simulink model "HevP2PowertrainController"  (R2022a)
settings: Solver=FixedStepDiscrete  StartTime=0  StopTime=inf  FixedStep=0.01  RelTol=1e-3  EnableMultiTasking=on
model workspace (MAT data in the model file):
  BattChargeMax = Simulink.Parameter
  BattChargeMax.Value = 5.3
  BattChargeMax.DataType = 'double'
  BattChargeMax.Complexity = 'real'
  BattChargeMax.Dimensions = [1 1]
  BattChrgPwrMax = Simulink.Parameter
  BattChrgPwrMax.Value = -30000
  BattChrgPwrMax.DataType = 'double'
  BattChrgPwrMax.Complexity = 'real'
  BattChrgPwrMax.Dimensions = [1 1]
  BattDischrgPwrMax = Simulink.Parameter
  BattDischrgPwrMax.Value = 46000
  BattDischrgPwrMax.DataType = 'double'
  BattDischrgPwrMax.Complexity = 'real'
  BattDischrgPwrMax.Dimensions = [1 1]
  BattEnrgy = Simulink.Parameter
  BattEnrgy.Value = 5724000
  BattEnrgy.DataType = 'double'
  BattEnrgy.Complexity = 'real'
  BattEnrgy.Dimensions = [1 1]
  BrkPrsMax = Simulink.Parameter
  BrkPrsMax.Value = 8300000
  BrkPrsMax.DataType = 'double'
  BrkPrsMax.Complexity = 'real'
  BrkPrsMax.Dimensions = [1 1]
  CSChrgFctr = Simulink.Parameter
  CSChrgFctr.Value = 0.2337
  CSChrgFctr.DataType = 'double'
  CSChrgFctr.Complexity = 'real'
  CSChrgFctr.Dimensions = [1 1]
  ChrgLmt_bpt = Simulink.Parameter
  ChrgLmt_bpt.Value = [1 1 1 1 1 1 1 1 0.7 0.35 0]
  ChrgLmt_bpt.DataType = 'double'
  ChrgLmt_bpt.Complexity = 'real'
  ChrgLmt_bpt.Dimensions = [1 11]
  DischrgLmt_bpt = Simulink.Parameter
  DischrgLmt_bpt.Value = [0 0.35 0.7 1 1 1 1 1 1 1 1]
  DischrgLmt_bpt.DataType = 'double'
  DischrgLmt_bpt.Complexity = 'real'
  DischrgLmt_bpt.Dimensions = [1 11]
  EVSpdLmt = Simulink.Parameter
  EVSpdLmt.Value = 17.9
  EVSpdLmt.DataType = 'double'
  EVSpdLmt.Complexity = 'real'
  EVSpdLmt.Dimensions = [1 1]
  EngIdle = Simulink.Parameter
  EngIdle.Value = 78.5398163397
  EngIdle.DataType = 'double'
  EngIdle.Complexity = 'real'
  EngIdle.Dimensions = [1 1]
  EngPwr = Simulink.Parameter
  EngPwr.Value = [1000 7500 15052.6315789 19736.8421053 24421.0526316 29105.2631579 33789.4736842 38473.6842105 43157.8947368 47842.1052632 52526.3157895 57210.5263158 61894.7368421 66578.9473684 71263.1578947 75947.3684211 80631.5789474 85315.7894737 90000]
  EngPwr.DataType = 'double'
  EngPwr.Complexity = 'real'
  EngPwr.Dimensions = [1 19]
  EngPwr_min = Simulink.Parameter
  EngPwr_min.Value = 11408
  EngPwr_min.DataType = 'double'
  EngPwr_min.Complexity = 'real'
  EngPwr_min.Dimensions = [1 1]
  EngSpd = Simulink.Parameter
  EngSpd.Value = [1000 1200 1448.84862461 1712.99052669 1980.33600187 2249.1155588 2517.55970613 2783.89895252 3046.3638066 3303.18477703 3552.59237246 3792.81710154 4022.08947291 4238.63999523 4440.69917715 4626.49752731 4794.26555436 4942.23376695 5068.63267374]
  EngSpd.DataType = 'double'
  EngSpd.Complexity = 'real'
  EngSpd.Dimensions = [1 19]
  EngSpdStart = Simulink.Parameter
  EngSpdStart.Value = 20
  EngSpdStart.DataType = 'double'
  EngSpdStart.Complexity = 'real'
  EngSpdStart.Dimensions = [1 1]
  EngTrq = Simulink.Parameter
  EngTrq.Value = [9.54929658551 59.6831036595 99.2112225513 110.02568665 117.759751017 123.57514891 128.166058939 131.971967205 135.285068696 138.308475993 141.18967656 144.040766791 146.951280713 149.9967243 153.244568751 156.75874496 160.603298419 164.845657961 169.559869104]
  EngTrq.DataType = 'double'
  EngTrq.Complexity = 'real'
  EngTrq.Dimensions = [1 19]
  MotTrq = Simulink.Parameter
  MotTrq.Value = [200 200 200 200 190.9859317 143.2394488 114.591559 95.49296586 81.85111359 71.61972439 63.66197724 57.29577951 52.08707228 47.74648293]
  MotTrq.DataType = 'double'
  MotTrq.Complexity = 'real'
  MotTrq.Dimensions = [1 14]
  N = Simulink.Parameter
  N.Value = [1 4.212 2.637 1.8 1.386 1 0.772]
  N.DataType = 'double'
  N.Complexity = 'real'
  N.Dimensions = [1 7]
  Ndiff = Simulink.Parameter
  Ndiff.Value = 3.32
  Ndiff.DataType = 'double'
  Ndiff.Complexity = 'real'
  Ndiff.Dimensions = [1 1]
  RegenBrkCutOff = Simulink.Parameter
  RegenBrkCutOff.Value = [0 1]
  RegenBrkCutOff.DataType = 'double'
  RegenBrkCutOff.Complexity = 'real'
  RegenBrkCutOff.Dimensions = [1 2]
  RegenBrkSpd_bpt = Simulink.Parameter
  RegenBrkSpd_bpt.Value = [5 9]
  RegenBrkSpd_bpt.DataType = 'double'
  RegenBrkSpd_bpt.Complexity = 'real'
  RegenBrkSpd_bpt.Dimensions = [1 2]
  Rm = Simulink.Parameter
  Rm.Value = 0.15
  Rm.DataType = 'double'
  Rm.Complexity = 'real'
  Rm.Dimensions = [1 1]
  SOCChrgFctr = Simulink.Parameter
  SOCChrgFctr.Value = 17969
  SOCChrgFctr.DataType = 'double'
  SOCChrgFctr.Complexity = 'real'
  SOCChrgFctr.Dimensions = [1 1]
  SOCChrgFctr_SOC_bpt = Simulink.Parameter
  SOCChrgFctr_SOC_bpt.Value = [50 60]
  SOCChrgFctr_SOC_bpt.DataType = 'double'
  SOCChrgFctr_SOC_bpt.Complexity = 'real'
  SOCChrgFctr_SOC_bpt.Dimensions = [1 2]
  SOCChrgFctr_VehSpd_bpt = Simulink.Parameter
  SOCChrgFctr_VehSpd_bpt.Value = [2.2352 10]
  SOCChrgFctr_VehSpd_bpt.DataType = 'double'
  SOCChrgFctr_VehSpd_bpt.Complexity = 'real'
  SOCChrgFctr_VehSpd_bpt.Dimensions = [1 2]
  SOCTrgt = Simulink.Parameter
  SOCTrgt.Value = 60
  SOCTrgt.DataType = 'double'
  SOCTrgt.Complexity = 'real'
  SOCTrgt.Dimensions = [1 1]
  SOC_bpt = Simulink.Parameter
  SOC_bpt.Value = [0 10 20 30 40 50 60 70 80 90 100]
  SOC_bpt.DataType = 'double'
  SOC_bpt.Complexity = 'real'
  SOC_bpt.Dimensions = [1 11]
  SOCmin = Simulink.Parameter
  SOCmin.Value = 50
  SOCmin.DataType = 'double'
  SOCmin.Complexity = 'real'
  SOCmin.Dimensions = [1 1]
  T_eff_bp = Simulink.Parameter
  T_eff_bp.Value = [0 20 40 60 80 100 120 140 160 180 200]
  T_eff_bp.DataType = 'double'
  T_eff_bp.Complexity = 'real'
  T_eff_bp.Dimensions = [1 11]
  VehMass = Simulink.Parameter
  VehMass.Value = 1623
  VehMass.DataType = 'double'
  VehMass.Complexity = 'real'
  VehMass.Dimensions = [1 1]
  disk_abore = Simulink.Parameter
  disk_abore.Value = 0.05
  disk_abore.DataType = 'double'
  disk_abore.Complexity = 'real'
  disk_abore.Dimensions = [1 1]
  efficiency_table = Simulink.Parameter
  efficiency_table.Value = [52  78  80  82  82  80  78  78  76  74  70; 52  78  80  82  82  80  78  78  76  74  70; 52  78  84  86  86  86  86  84  84  82  82; 52  80  86  86  88  88  88  86  86  84  84; 52  80  86  88  88  88  88  88  86  86  86; 52  80  86  88  90  90  90  90  88  88  88; 52  82  88  90  91  91  92  92  92  91  91; 52  82  88  91  91  92  93  93  93  93  93; 52  84  90  92  92  93  93  93  93  93  93; 62  86  91  93  93  93  93  93  93  93  93; 66  86  91  93  93  93  93  93  93  93  93; 70  86  92  93  93  93  93  93  93  93  93; 70  86  92  93  93  93  93  93  93  93  93; 72  86  91  93  93  93  93  93  93  93  93]
  efficiency_table.DataType = 'double'
  efficiency_table.Complexity = 'real'
  efficiency_table.Dimensions = [14 11]
  mu_kinetic = Simulink.Parameter
  mu_kinetic.Value = 0.35
  mu_kinetic.DataType = 'double'
  mu_kinetic.Complexity = 'real'
  mu_kinetic.Dimensions = [1 1]
  num_pads = Simulink.Parameter
  num_pads.Value = 2
  num_pads.DataType = 'double'
  num_pads.Complexity = 'real'
  num_pads.Dimensions = [1 1]
  w_eff_bp = Simulink.Parameter
  w_eff_bp.Value = [0 500 1000 1432.391138 1500 2000 2500 3000 3500 4000 4500 5000 5500 6000]
  w_eff_bp.DataType = 'double'
  w_eff_bp.Complexity = 'real'
  w_eff_bp.Dimensions = [1 14]
libraries: simulink x7, autolibutils x1, autolibhevctrlrcommon x1
settings Model: DataDictionary=HevP2PowertrainController.sldd  ModifiedByFormat=The MathWorks, Inc.  Creator=The MathWorks, Inc.  LastModifiedBy=The MathWorks, Inc.
settings SolverCC: AlgebraicLoopSolver=TrustRegion  AutoInsertRateTranBlk=on  MaxZcPerStep=1
settings DataIOCC: SaveOutput=off  SignalLogging=off  DSMLogging=off  SaveTime=off  ReturnWorkspaceOutputs=off
settings OptimizationCC: EfficientMapNaN2IntZero=off
settings DebuggingCC: UnderspecifiedInitializationDetection=Classic  MergeDetectMultiDrivingBlocksExec=none  UnconnectedInputMsg=warning  UnconnectedOutputMsg=warning  UnconnectedLineMsg=warning  SFUnusedDataAndEventsDiag=none  SFMachineParentedDataDiag=warning  ArithmeticOperatorsInVariantConditions=warning
settings HardwareCC: TargetBitPerLong=64  TargetBitPerPointer=64  TargetBitPerSizeT=64  TargetBitPerPtrDiffT=64  TargetLongLongMode=on  TargetIntDivRoundTo=Zero  TargetEndianess=LittleEndian  TargetWordSize=64  TargetHWDeviceType=MATLAB Host  ProdEqTarget=off
settings SFSimCC: SimUseLocalCustomCode=off  CustomCodeUndefinedFunction=UseInterfaceOnly
settings RTWCC: RTWUseLocalCustomCode=off  DLArmComputeVersion=19.05
settings CodeAppCC: MaxIdLength=128  StateflowObjectComments=on
settings GRTTargetCC: TargetLangStandard=C89/C90 (ANSI)  CombineOutputUpdateFcns=off  GRTInterface=on
settings ConfigComp: CovMetricSettings=dsw  CovSaveCumulativeToWorkspaceVar=on  CovSaveSingleToWorkspaceVar=on  CovExternalEMLEnable=off

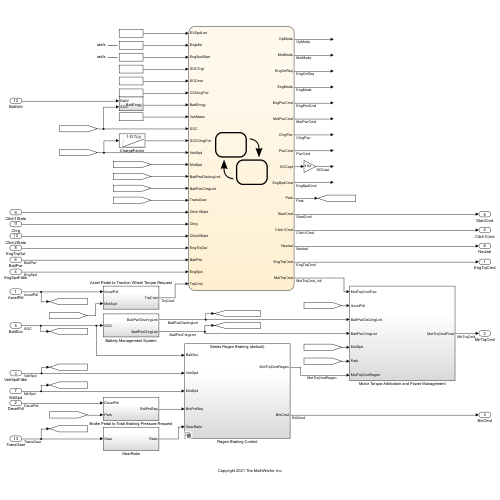
[thumbnail: Simulink's stored preview of the top-level diagram]
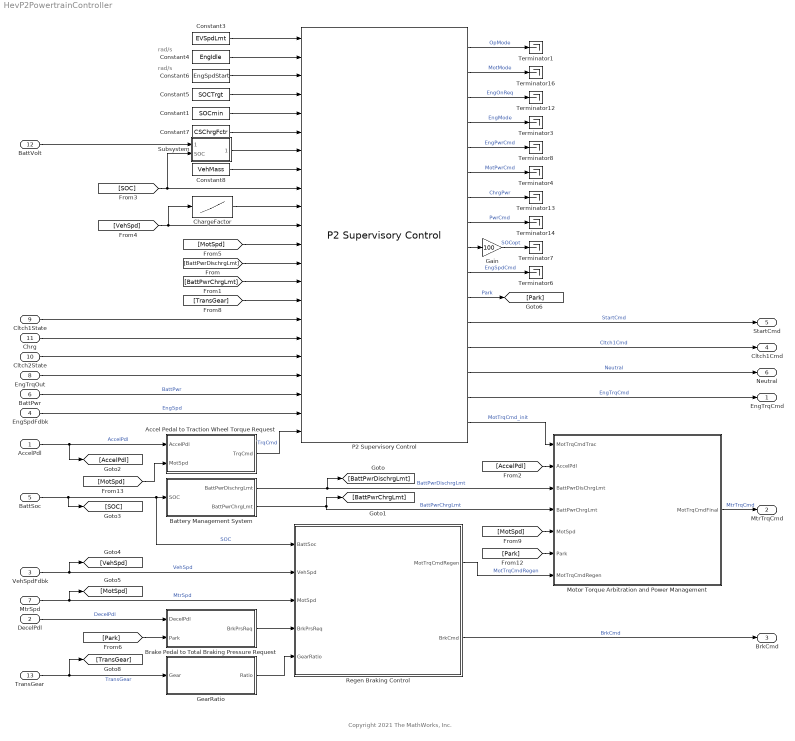
== system HevP2PowertrainController ==
  note: rad/s
  note: rad/s
  note: Copyright 2021 The MathWorks, Inc.
  AccelPdl : Inport  OutDataTypeStr=double  PortDimensions=1  SampleTime=[0.01,0]
  DecelPdl : Inport  Port=2  OutDataTypeStr=double  PortDimensions=1  SampleTime=[0.01,0]
  VehSpdFdbk : Inport  Port=3  OutDataTypeStr=double  PortDimensions=1  SampleTime=[0.01,0]
  EngSpdFdbk : Inport  Port=4  OutDataTypeStr=double  PortDimensions=1  SampleTime=[0.01,0]
  BattSoc : Inport  Port=5  OutDataTypeStr=double  PortDimensions=1  SampleTime=[0.01,0]
  BattPwr : Inport  Port=6  OutDataTypeStr=double  PortDimensions=1  SampleTime=[0.01,0]
  MtrSpd : Inport  Port=7  OutDataTypeStr=double  PortDimensions=1  SampleTime=[0.01,0]
  EngTrqOut : Inport  Port=8  OutDataTypeStr=double  PortDimensions=1  SampleTime=[0.01,0]
  Cltch1State : Inport  Port=9  OutDataTypeStr=boolean  PortDimensions=1  SampleTime=[0.01,0]
  Cltch2State : Inport  Port=10  OutDataTypeStr=boolean  PortDimensions=1  SampleTime=[0.01,0]
  Chrg : Inport  Port=11  OutDataTypeStr=boolean  PortDimensions=1  SampleTime=[0.01,0]
  BattVolt : Inport  Port=12  OutDataTypeStr=double  PortDimensions=1  SampleTime=[0.01,0]
  TransGear : Inport  Port=13  OutDataTypeStr=double  PortDimensions=1  SampleTime=[0.01,0]
  Accel Pedal to Traction Wheel Torque Request : Subsystem
  Battery Management System : Subsystem
  Brake Pedal to Total Braking Pressure Request : Subsystem
  ChargeFactor : Lookup_n-D  NumberOfTableDimensions=1  BreakpointsForDimension1=SOCChrgFctr_VehSpd_bpt  BreakpointsForDimension2=SOCChrgFctr_VehSpd_bpt  Table=[0 SOCChrgFctr]  ExtrapMethod=Clip  UseLastTableValue=on  InternalRulePriority=Speed  RndMeth=Simplest
  Constant1 : Constant  Value=SOCmin
  Constant3 : Constant  Value=EVSpdLmt
  Constant4 : Constant  Value=EngIdle
  Constant5 : Constant  Value=SOCTrgt
  Constant6 : Constant  Value=EngSpdStart
  Constant7 : Constant  Value=CSChrgFctr
  Constant8 : Constant  Value=VehMass
  Gain : Gain  Gain=100
  GearRatio : Subsystem
  Motor Torque Arbitration and Power Management : Subsystem
  P2 Supervisory Control : autolibhevctrlrcommon/P2 Supervisory Control  aMode=1
      settings: SourceProductBaseCode=PW
  Regen Braking Control : Subsystem  Variant=on  VariantControlMode=label  VariantControl=(default)  LabelModeActiveChoice=(default)
  Subsystem : Subsystem
  Terminator{1,3..4,6..8,12..14,16} (10 alike) : Terminator
  EngTrqCmd : Outport  OutDataTypeStr=double  PortDimensions=1  SampleTime=[0.01,0]  VectorParamsAs1DForOutWhenUnconnected=off
  MtrTrqCmd : Outport  Port=2  OutDataTypeStr=double  PortDimensions=1  SampleTime=[0.01,0]  VectorParamsAs1DForOutWhenUnconnected=off
  BrkCmd : Outport  Port=3  OutDataTypeStr=double  PortDimensions=1  SampleTime=[0.01,0]  VectorParamsAs1DForOutWhenUnconnected=off
  Cltch1Cmd : Outport  Port=4  PortDimensions=1  SampleTime=[0.01,0]  VectorParamsAs1DForOutWhenUnconnected=off
  StartCmd : Outport  Port=5  PortDimensions=1  SampleTime=[0.01,0]  VectorParamsAs1DForOutWhenUnconnected=off
  Neutral : Outport  Port=6  PortDimensions=1  SampleTime=[0.01,0]  VectorParamsAs1DForOutWhenUnconnected=off
  wires:
  AccelPdl/1 -> [AccelPdl], Accel Pedal to Traction Wheel Torque Request/1(AccelPdl)  "AccelPdl"
  DecelPdl/1 -> Brake Pedal to Total Braking Pressure Request/1(DecelPdl)  "DecelPdl"
  VehSpdFdbk/1 -> [VehSpd], Regen Braking Control/2("VehSpd ")  "VehSpd"
  EngSpdFdbk/1 -> P2 Supervisory Control/21  "EngSpd"
  BattPwr/1 -> P2 Supervisory Control/20  "BattPwr"
  BattSoc/1 -> [SOC], Regen Braking Control/1("BattSoc "), Battery Management System/1(SOC)  "SOC"
  MtrSpd/1 -> [MotSpd], Regen Braking Control/3("MotSpd ")  "MtrSpd"
  Battery Management System/2(BattPwrChrgLmt) -> [BattPwrChrgLmt], Motor Torque Arbitration and Power Management/4("BattPwrChrgLmt ")  "BattPwrChrgLmt"
  Battery Management System/1(BattPwrDischrgLmt) -> [BattPwrDischrgLmt], Motor Torque Arbitration and Power Management/3(BattPwrDisChrgLmt)  "BattPwrDischrgLmt"
  P2 Supervisory Control/1 -> Terminator1/1  "OpMode"
  P2 Supervisory Control/5 -> Terminator8/1  "EngPwrCmd"
  P2 Supervisory Control/3 -> Terminator12/1  "EngOnReq"
  P2 Supervisory Control/6 -> Terminator4/1  "MotPwrCmd"
  [SOC] -> P2 Supervisory Control/9, Subsystem/2(SOC)
  [VehSpd] -> P2 Supervisory Control/11, ChargeFactor/1
  Constant3/1 -> P2 Supervisory Control/1
  [BattPwrDischrgLmt] -> P2 Supervisory Control/13
  [BattPwrChrgLmt] -> P2 Supervisory Control/14
  Accel Pedal to Traction Wheel Torque Request/1(TrqCmd) -> P2 Supervisory Control/22  "TrqCmd"
  Constant4/1 -> P2 Supervisory Control/2
  P2 Supervisory Control/16 -> Motor Torque Arbitration and Power Management/1(MotTrqCmdTrac)  "MotTrqCmd_init"
  Brake Pedal to Total Braking Pressure Request/1(BrkPrsReq) -> Regen Braking Control/4("BrkPrsReq ")
  Regen Braking Control/1(" MotTrqCmdRegen") -> Motor Torque Arbitration and Power Management/7(MotTrqCmdRegen)  "MotTrqCmdRegen"
  Regen Braking Control/2(" BrkCmd") -> BrkCmd/1  "BrkCmd"
  P2 Supervisory Control/9 -> Gain/1
  P2 Supervisory Control/7 -> Terminator13/1  "ChrgPwr"
  P2 Supervisory Control/8 -> Terminator14/1  "PwrCmd"
  [MotSpd] -> P2 Supervisory Control/12
  Gain/1 -> Terminator7/1  "SOCopt"
  P2 Supervisory Control/4 -> Terminator3/1  "EngMode"
  P2 Supervisory Control/10 -> Terminator6/1  "EngSpdCmd"
  P2 Supervisory Control/2 -> Terminator16/1  "MotMode"
  Constant5/1 -> P2 Supervisory Control/4
  [AccelPdl] -> Motor Torque Arbitration and Power Management/2(AccelPdl)
  Motor Torque Arbitration and Power Management/1(MotTrqCmdFinal) -> MtrTrqCmd/1  "MtrTrqCmd"
  Constant1/1 -> P2 Supervisory Control/5
  P2 Supervisory Control/15 -> EngTrqCmd/1  "EngTrqCmd"
  EngTrqOut/1 -> P2 Supervisory Control/19
  P2 Supervisory Control/11 -> [Park]  "Park"
  [Park] -> Brake Pedal to Total Braking Pressure Request/2(Park)
  [MotSpd] -> Motor Torque Arbitration and Power Management/5(MotSpd)
  GearRatio/1(Ratio) -> Regen Braking Control/5(GearRatio)
  TransGear/1 -> [TransGear], GearRatio/1(Gear)  "TransGear"
  P2 Supervisory Control/13 -> Cltch1Cmd/1  "Cltch1Cmd"
  Cltch2State/1 -> P2 Supervisory Control/18
  Cltch1State/1 -> P2 Supervisory Control/16
  P2 Supervisory Control/14 -> Neutral/1  "Neutral"
  [Park] -> Motor Torque Arbitration and Power Management/6(Park)
  [MotSpd] -> Accel Pedal to Traction Wheel Torque Request/2(MotSpd)
  P2 Supervisory Control/12 -> StartCmd/1  "StartCmd"
  ChargeFactor/1 -> P2 Supervisory Control/10
  Chrg/1 -> P2 Supervisory Control/17
  Constant6/1 -> P2 Supervisory Control/3
  Subsystem/1(BattEnrgy) -> P2 Supervisory Control/7
  Constant8/1 -> P2 Supervisory Control/8
  [TransGear] -> P2 Supervisory Control/15
  BattVolt/1 -> Subsystem/1(BattV)
  Constant7/1 -> P2 Supervisory Control/6

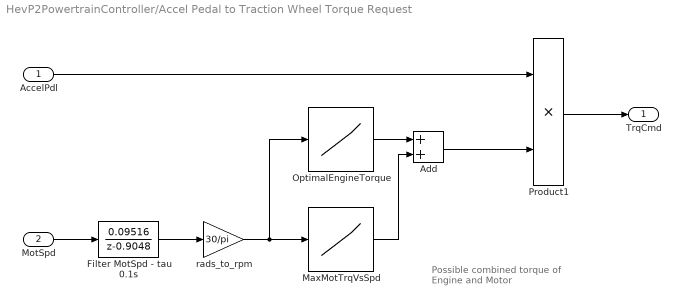
== system HevP2PowertrainController/Accel Pedal to Traction Wheel Torque Request ==
  note: Possible combined torque
      | of Engine and Motor
  AccelPdl : Inport
  MotSpd : Inport  Port=2
  Add : Sum
  Filter MotSpd - tau 0.1s : DiscreteTransferFcn  Numerator=[0.09516]  Denominator=[1 -0.9048]
  MaxMotTrqVsSpd : Lookup_n-D  NumberOfTableDimensions=1  BreakpointsForDimension1=w_eff_bp  Table=MotTrq  ExtrapMethod=Clip  UseLastTableValue=on  InternalRulePriority=Speed  OutDataTypeStr=Inherit: Inherit from 'Table data'  RndMeth=Simplest
  OptimalEngineTorque : Lookup_n-D  NumberOfTableDimensions=1  BreakpointsForDimension1=[0 EngSpd]  Table=[0 EngTrq]  ExtrapMethod=Clip  UseLastTableValue=on  InternalRulePriority=Speed  RndMeth=Simplest
  Product1 : Product
  rads_to_rpm : Gain  Gain=30/pi
  TrqCmd : Outport  VectorParamsAs1DForOutWhenUnconnected=off
  wires:
  Product1/1 -> TrqCmd/1
  Add/1 -> Product1/2
  AccelPdl/1 -> Product1/1
  MotSpd/1 -> Filter MotSpd - tau 0.1s/1
  OptimalEngineTorque/1 -> Add/1
  MaxMotTrqVsSpd/1 -> Add/2
  rads_to_rpm/1 -> OptimalEngineTorque/1, MaxMotTrqVsSpd/1
  Filter MotSpd - tau 0.1s/1 -> rads_to_rpm/1

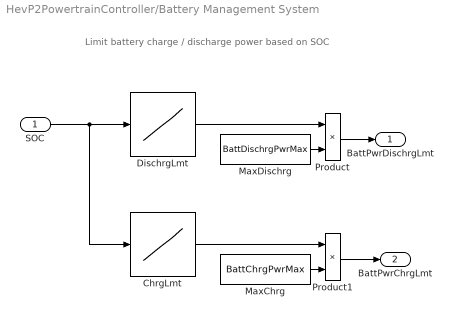
== system HevP2PowertrainController/Battery Management System ==
  note: Limit battery charge / discharge power based on SOC
  SOC : Inport
  ChrgLmt : Lookup_n-D  NumberOfTableDimensions=1  BreakpointsForDimension1=SOC_bpt  Table=ChrgLmt_bpt  ExtrapMethod=Clip  UseLastTableValue=on  InternalRulePriority=Speed  RndMeth=Simplest
  DischrgLmt : Lookup_n-D  NumberOfTableDimensions=1  BreakpointsForDimension1=SOC_bpt  Table=DischrgLmt_bpt  ExtrapMethod=Clip  UseLastTableValue=on  InternalRulePriority=Speed  RndMeth=Simplest
  MaxChrg : Constant  Value=BattChrgPwrMax
  MaxDischrg : Constant  Value=BattDischrgPwrMax
  Product : Product
  Product1 : Product
  BattPwrDischrgLmt : Outport  VectorParamsAs1DForOutWhenUnconnected=off
  BattPwrChrgLmt : Outport  Port=2  VectorParamsAs1DForOutWhenUnconnected=off
  wires:
  SOC/1 -> DischrgLmt/1, ChrgLmt/1
  MaxChrg/1 -> Product1/2
  MaxDischrg/1 -> Product/2
  Product/1 -> BattPwrDischrgLmt/1
  Product1/1 -> BattPwrChrgLmt/1
  ChrgLmt/1 -> Product1/1
  DischrgLmt/1 -> Product/1

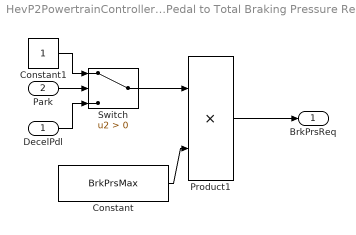
== system HevP2PowertrainController/Brake Pedal to Total Braking Pressure Request ==
  DecelPdl : Inport
  Park : Inport  Port=2
  Constant : Constant  Value=BrkPrsMax
  Constant1 : Constant
  Product1 : Product
  Switch : Switch  Criteria=u2 > Threshold  SaturateOnIntegerOverflow=off  InputSameDT=off
  BrkPrsReq : Outport  VectorParamsAs1DForOutWhenUnconnected=off
  wires:
  Constant/1 -> Product1/2
  Switch/1 -> Product1/1
  DecelPdl/1 -> Switch/3
  Constant1/1 -> Switch/1
  Product1/1 -> BrkPrsReq/1
  Park/1 -> Switch/2

== system HevP2PowertrainController/GearRatio ==
  Gear : Inport
  Gain : Gain  Gain=Ndiff
  Multiport Switch : MultiPortSwitch  DataPortOrder=Zero-based contiguous  Inputs=1  zeroidx=on  SaturateOnIntegerOverflow=off  InputSameDT=off
  Trans Gear Ratios : Constant  Value=N
  Ratio : Outport  VectorParamsAs1DForOutWhenUnconnected=off
  wires:
  Gear/1 -> Multiport Switch/1
  Multiport Switch/1 -> Gain/1
  Gain/1 -> Ratio/1
  Trans Gear Ratios/1 -> Multiport Switch/2

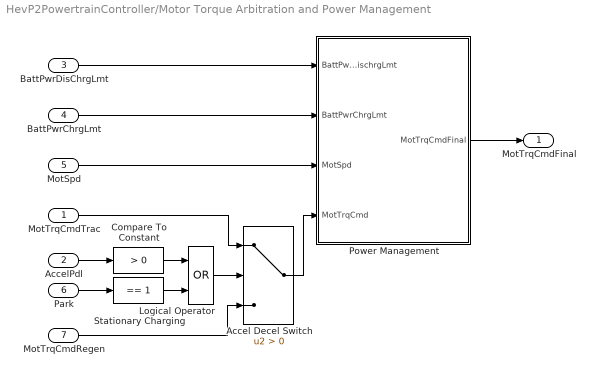
== system HevP2PowertrainController/Motor Torque Arbitration and Power Management ==
  MotTrqCmdTrac : Inport
  AccelPdl : Inport  Port=2
  BattPwrDisChrgLmt : Inport  Port=3
  "BattPwrChrgLmt " : Inport  Port=4
  MotSpd : Inport  Port=5
  Park : Inport  Port=6
  MotTrqCmdRegen : Inport  Port=7
  Accel Decel Switch : Switch  Criteria=u2 > Threshold  SaturateOnIntegerOverflow=off  InputSameDT=off
  Compare To Constant : simulink/Logic and Bit Operations/Compare To Constant  relop=>  const=0  OutDataTypeStr=boolean
  Logical Operator : Logic  Operator=OR  AllPortsSameDT=off  OutDataTypeStr=boolean
  Power Management : Subsystem
  Stationary Charging : simulink/Logic and Bit Operations/Compare To Constant  relop===  const=1  OutDataTypeStr=boolean
  MotTrqCmdFinal : Outport  VectorParamsAs1DForOutWhenUnconnected=off
  wires:
  AccelPdl/1 -> Compare To Constant/1
  MotTrqCmdTrac/1 -> Accel Decel Switch/1
  Power Management/1(MotTrqCmdFinal) -> MotTrqCmdFinal/1
  Accel Decel Switch/1 -> Power Management/4(MotTrqCmd)
  BattPwrDisChrgLmt/1 -> Power Management/1(BattPwrDischrgLmt)
  "BattPwrChrgLmt "/1 -> Power Management/2(BattPwrChrgLmt)
  MotSpd/1 -> Power Management/3(MotSpd)
  Compare To Constant/1 -> Logical Operator/1
  Stationary Charging/1 -> Logical Operator/2
  Logical Operator/1 -> Accel Decel Switch/2
  Park/1 -> Stationary Charging/1
  MotTrqCmdRegen/1 -> Accel Decel Switch/3

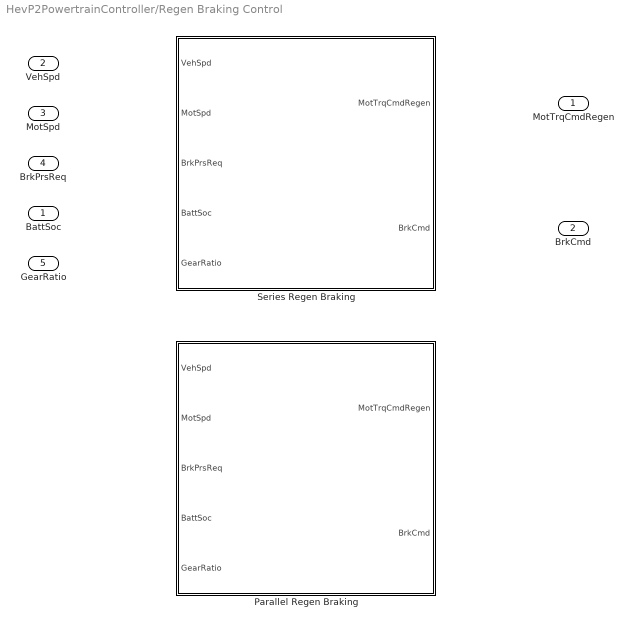
== system HevP2PowertrainController/Regen Braking Control ==
  "BattSoc " : Inport
  "VehSpd " : Inport  Port=2
  "MotSpd " : Inport  Port=3
  "BrkPrsReq " : Inport  Port=4
  GearRatio : Inport  Port=5
  Parallel Regen Braking : Subsystem  VariantControl=Variant
  Series Regen Braking : Subsystem  VariantControl=(default)
  " MotTrqCmdRegen" : Outport  VectorParamsAs1DForOutWhenUnconnected=off
  " BrkCmd" : Outport  Port=2  VectorParamsAs1DForOutWhenUnconnected=off

== system HevP2PowertrainController/Subsystem ==
  BattV : Inport
  SOC : Inport  Port=2
  BattCap_As : Constant  Value=BattChargeMax*3600
  Gain1 : Gain  Gain=1/100
  Product : Product  Inputs=3
  BattEnrgy : Outport  VectorParamsAs1DForOutWhenUnconnected=off
  wires:
  SOC/1 -> Gain1/1
  Gain1/1 -> Product/3
  BattV/1 -> Product/2
  BattCap_As/1 -> Product/1
  Product/1 -> BattEnrgy/1

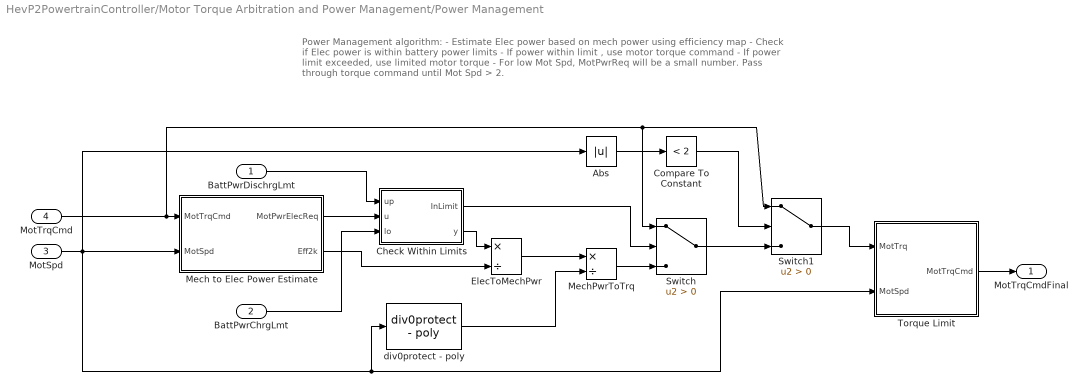
== system HevP2PowertrainController/Motor Torque Arbitration and Power Management/Power Management ==
  note: Power Management algorithm:
      | - Estimate Elec power based on mech power using efficiency map
      | - Check if Elec power is within battery power limits
      | - If power within limit , use motor torque command
      | - If power limit exceeded, use limited motor torque
      | - For low Mot Spd, MotPwrReq will be a small number.  Pass through torque command until Mot Spd > 2.
  BattPwrDischrgLmt : Inport
  BattPwrChrgLmt : Inport  Port=2
  MotSpd : Inport  Port=3
  MotTrqCmd : Inport  Port=4
  Abs : Abs  SaturateOnIntegerOverflow=off
  Check Within Limits : Subsystem
  Compare To Constant : simulink/Logic and Bit Operations/Compare To Constant  relop=<  const=2  OutDataTypeStr=boolean
  ElecToMechPwr : Product  Inputs=*/
  Mech to Elec Power Estimate : Subsystem
  MechPwrToTrq : Product  Inputs=*/
  Switch : Switch  Criteria=u2 > Threshold  SaturateOnIntegerOverflow=off  InputSameDT=off
  Switch1 : Switch  Criteria=u2 > Threshold  SaturateOnIntegerOverflow=off  InputSameDT=off
  Torque Limit : Subsystem
  div0protect - poly : autolibutils/div0protect - poly  thresh=2  ZeroCross1=off  aMode=aMode
      settings: SourceProductBaseCode=PW,DR,MT,VE
  MotTrqCmdFinal : Outport  VectorParamsAs1DForOutWhenUnconnected=off
  wires:
  MotSpd/1 -> Abs/1, Torque Limit/2(MotSpd), div0protect - poly/1, Mech to Elec Power Estimate/2(MotSpd)
  MotTrqCmd/1 -> Switch/1, Switch1/1, Mech to Elec Power Estimate/1(MotTrqCmd)
  div0protect - poly/1 -> MechPwrToTrq/2
  Mech to Elec Power Estimate/2(Eff2k) -> ElecToMechPwr/2
  ElecToMechPwr/1 -> MechPwrToTrq/1
  MechPwrToTrq/1 -> Switch/3
  Torque Limit/1(MotTrqCmd) -> MotTrqCmdFinal/1
  BattPwrDischrgLmt/1 -> Check Within Limits/1(up)
  Mech to Elec Power Estimate/1(MotPwrElecReq) -> Check Within Limits/2(u)
  BattPwrChrgLmt/1 -> Check Within Limits/3(lo)
  Check Within Limits/2(y) -> ElecToMechPwr/1
  Switch/1 -> Switch1/3
  Check Within Limits/1(InLimit) -> Switch/2
  Switch1/1 -> Torque Limit/1(MotTrq)
  Abs/1 -> Compare To Constant/1
  Compare To Constant/1 -> Switch1/2

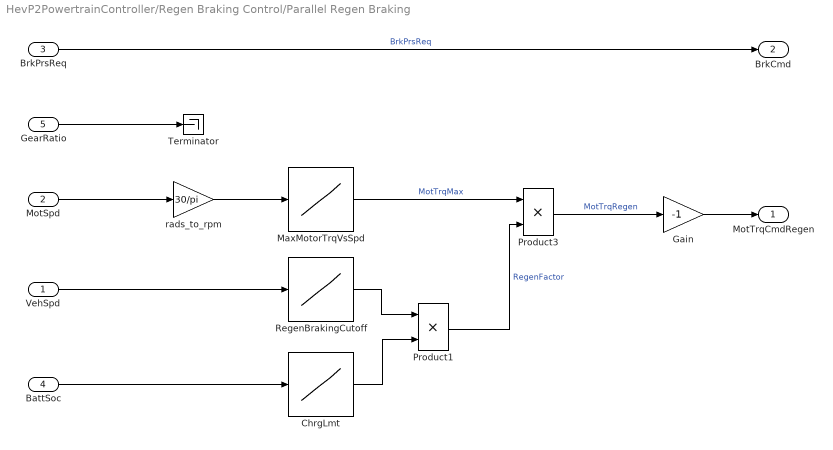
== system HevP2PowertrainController/Regen Braking Control/Parallel Regen Braking ==
  VehSpd : Inport
  MotSpd : Inport  Port=2
  "BrkPrsReq " : Inport  Port=3
  BattSoc : Inport  Port=4
  GearRatio : Inport  Port=5
  ChrgLmt : Lookup_n-D  NumberOfTableDimensions=1  BreakpointsForDimension1=SOC_bpt  Table=ChrgLmt_bpt  ExtrapMethod=Clip  UseLastTableValue=on  InternalRulePriority=Speed  RndMeth=Simplest
  Gain : Gain  Gain=-1
  MaxMotorTrqVsSpd : Lookup_n-D  NumberOfTableDimensions=1  BreakpointsForDimension1=w_eff_bp  Table=MotTrq  ExtrapMethod=Clip  UseLastTableValue=on  InternalRulePriority=Speed  OutDataTypeStr=Inherit: Inherit from 'Table data'  RndMeth=Simplest
  Product1 : Product
  Product3 : Product
  RegenBrakingCutoff : Lookup_n-D  NumberOfTableDimensions=1  BreakpointsForDimension1=RegenBrkSpd_bpt  Table=RegenBrkCutOff  ExtrapMethod=Clip  UseLastTableValue=on  InternalRulePriority=Speed  RndMeth=Simplest
  Terminator : Terminator
  rads_to_rpm : Gain  Gain=30/pi
  " MotTrqCmdRegen" : Outport  VectorParamsAs1DForOutWhenUnconnected=off
  " BrkCmd" : Outport  Port=2  VectorParamsAs1DForOutWhenUnconnected=off
  wires:
  Gain/1 -> " MotTrqCmdRegen"/1
  BattSoc/1 -> ChrgLmt/1
  Product3/1 -> Gain/1  "MotTrqRegen"
  Product1/1 -> Product3/2  "RegenFactor"
  RegenBrakingCutoff/1 -> Product1/1
  VehSpd/1 -> RegenBrakingCutoff/1
  ChrgLmt/1 -> Product1/2
  MaxMotorTrqVsSpd/1 -> Product3/1  "MotTrqMax"
  rads_to_rpm/1 -> MaxMotorTrqVsSpd/1
  MotSpd/1 -> rads_to_rpm/1
  "BrkPrsReq "/1 -> " BrkCmd"/1  "BrkPrsReq"
  GearRatio/1 -> Terminator/1

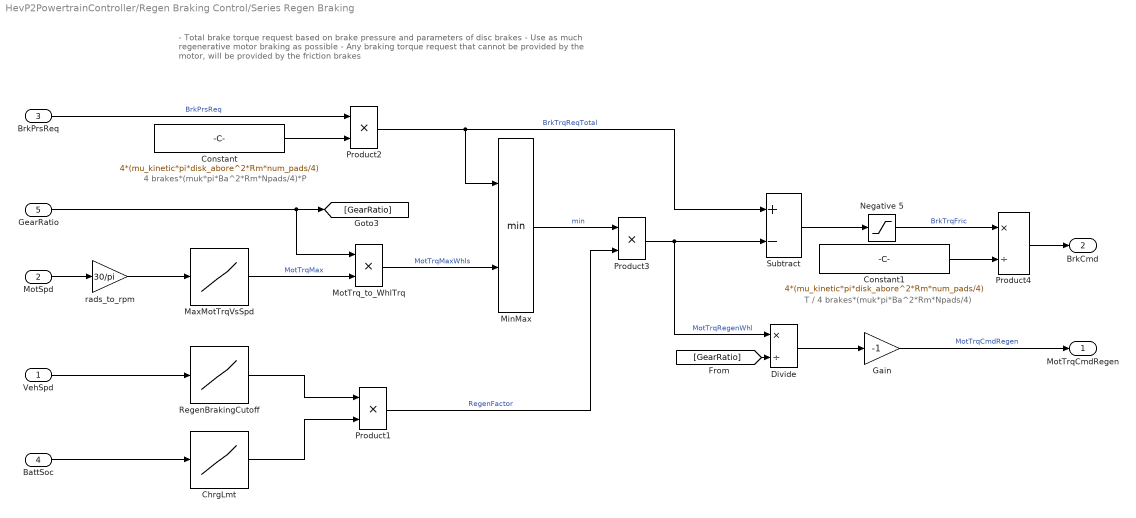
== system HevP2PowertrainController/Regen Braking Control/Series Regen Braking ==
  note: - Total brake torque request based on brake pressure and parameters of disc brakes
      | - Use as much regenerative motor braking as possible
      | -  Any braking torque request that cannot be provided by the motor, will be provided by the friction brakes
  note: T / 4 brakes*(muk*pi*Ba^2*Rm*Npads/4)
  note: 4 brakes*(muk*pi*Ba^2*Rm*Npads/4)*P
  VehSpd : Inport
  MotSpd : Inport  Port=2
  "BrkPrsReq " : Inport  Port=3
  BattSoc : Inport  Port=4
  GearRatio : Inport  Port=5
  ChrgLmt : Lookup_n-D  NumberOfTableDimensions=1  BreakpointsForDimension1=SOC_bpt  Table=ChrgLmt_bpt  ExtrapMethod=Clip  UseLastTableValue=on  InternalRulePriority=Speed  RndMeth=Simplest
  Constant : Constant  Value=4*(mu_kinetic*pi*disk_abore^2*Rm*num_pads/4)
  Constant1 : Constant  Value=4*(mu_kinetic*pi*disk_abore^2*Rm*num_pads/4)
  Divide : Product  Inputs=*/
  Gain : Gain  Gain=-1
  MaxMotTrqVsSpd : Lookup_n-D  NumberOfTableDimensions=1  BreakpointsForDimension1=w_eff_bp  Table=MotTrq  ExtrapMethod=Clip  UseLastTableValue=on  InternalRulePriority=Speed  OutDataTypeStr=Inherit: Inherit from 'Table data'  RndMeth=Simplest
  MinMax : MinMax  Inputs=2
  MotTrq_to_WhlTrq : Product
  Negative 5 : Saturate  UpperLimit=inf  LowerLimit=0
  Product1 : Product
  Product2 : Product
  Product3 : Product
  Product4 : Product  Inputs=*/
  RegenBrakingCutoff : Lookup_n-D  NumberOfTableDimensions=1  BreakpointsForDimension1=RegenBrkSpd_bpt  Table=RegenBrkCutOff  ExtrapMethod=Clip  UseLastTableValue=on  InternalRulePriority=Speed  RndMeth=Simplest
  Subtract : Sum  Inputs=+-
  rads_to_rpm : Gain  Gain=30/pi
  " MotTrqCmdRegen" : Outport  VectorParamsAs1DForOutWhenUnconnected=off
  " BrkCmd" : Outport  Port=2  VectorParamsAs1DForOutWhenUnconnected=off
  wires:
  Product3/1 -> Divide/1, Subtract/2  "MotTrqRegenWhl"
  Product4/1 -> " BrkCmd"/1
  Constant1/1 -> Product4/2
  Constant/1 -> Product2/2
  "BrkPrsReq "/1 -> Product2/1  "BrkPrsReq"
  rads_to_rpm/1 -> MaxMotTrqVsSpd/1
  MaxMotTrqVsSpd/1 -> MotTrq_to_WhlTrq/2  "MotTrqMax"
  Product2/1 -> MinMax/1, Subtract/1  "BrkTrqReqTotal"
  MinMax/1 -> Product3/1  "min"
  ChrgLmt/1 -> Product1/2
  VehSpd/1 -> RegenBrakingCutoff/1
  RegenBrakingCutoff/1 -> Product1/1
  Product1/1 -> Product3/2  "RegenFactor"
  Subtract/1 -> Negative 5/1
  BattSoc/1 -> ChrgLmt/1
  Negative 5/1 -> Product4/1  "BrkTrqFric"
  MotSpd/1 -> rads_to_rpm/1
  MotTrq_to_WhlTrq/1 -> MinMax/2  "MotTrqMaxWhls"
  Divide/1 -> Gain/1
  Gain/1 -> " MotTrqCmdRegen"/1  "MotTrqCmdRegen"
  GearRatio/1 -> [GearRatio], MotTrq_to_WhlTrq/1
  [GearRatio] -> Divide/2

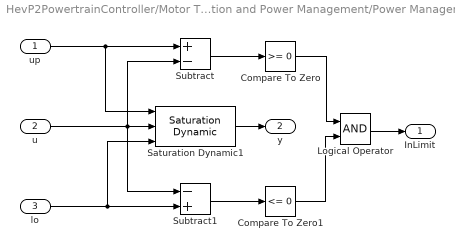
== system HevP2PowertrainController/Motor Torque Arbitration and Power Management/Power Management/Check Within Limits ==
  up : Inport
  u : Inport  Port=2
  lo : Inport  Port=3
  Compare To Zero : simulink/Logic and Bit Operations/Compare To Zero  relop=>=  OutDataTypeStr=boolean
  Compare To Zero1 : simulink/Logic and Bit Operations/Compare To Zero  relop=<=  OutDataTypeStr=boolean
  Logical Operator : Logic  AllPortsSameDT=off  OutDataTypeStr=boolean
  Saturation Dynamic1 : simulink/Discontinuities/Saturation Dynamic  OutMin=[]  OutMax=[]  OutDataTypeStr=Inherit: Same as second input  OutDataType=fixdt(1, 16)  OutScaling=2^-10  DoSatur=off
  Subtract : Sum  Inputs=+-
  Subtract1 : Sum  Inputs=-+
  InLimit : Outport  VectorParamsAs1DForOutWhenUnconnected=off
  y : Outport  Port=2  VectorParamsAs1DForOutWhenUnconnected=off
  wires:
  Saturation Dynamic1/1 -> y/1
  lo/1 -> Subtract1/2, Saturation Dynamic1/3
  up/1 -> Subtract/1, Saturation Dynamic1/1
  u/1 -> Subtract1/1, Subtract/2, Saturation Dynamic1/2
  Subtract/1 -> Compare To Zero/1
  Subtract1/1 -> Compare To Zero1/1
  Compare To Zero/1 -> Logical Operator/1
  Compare To Zero1/1 -> Logical Operator/2
  Logical Operator/1 -> InLimit/1

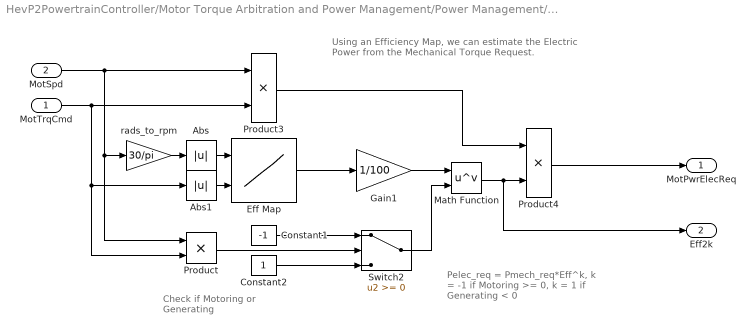
== system HevP2PowertrainController/Motor Torque Arbitration and Power Management/Power Management/Mech to Elec Power Estimate ==
  note: Check if Motoring
      | or Generating
  note: Using an Efficiency Map, we can estimate the
      | Electric Power from the Mechanical  Torque Request.
  note: Pelec_req = Pmech_req*Eff^k,
      | k = -1 if Motoring >= 0,
      | k = 1 if Generating < 0
  MotTrqCmd : Inport
  MotSpd : Inport  Port=2
  Abs : Abs  SaturateOnIntegerOverflow=off
  Abs1 : Abs  SaturateOnIntegerOverflow=off
  Constant1 : Constant  Value=-1  SampleTime=-1
  Constant2 : Constant  SampleTime=-1
  Eff Map : Lookup_n-D  BreakpointsForDimension1=w_eff_bp  BreakpointsForDimension2=T_eff_bp  Table=efficiency_table  ExtrapMethod=Clip  UseLastTableValue=on  InternalRulePriority=Speed  OutDataTypeStr=Inherit: Inherit from 'Table data'  RndMeth=Simplest
      settings: InputPortMap=u0,u1
  Gain1 : Gain  Gain=1/100
  Math Function : Math  Operator=pow  SignedPower=on  OutputSignalType=real
  Product : Product
  Product3 : Product
  Product4 : Product
  Switch2 : Switch  SaturateOnIntegerOverflow=off  InputSameDT=off
  rads_to_rpm : Gain  Gain=30/pi
  MotPwrElecReq : Outport  VectorParamsAs1DForOutWhenUnconnected=off
  Eff2k : Outport  Port=2  VectorParamsAs1DForOutWhenUnconnected=off
  wires:
  Product3/1 -> Product4/1
  Switch2/1 -> Math Function/2
  Constant1/1 -> Switch2/1
  Constant2/1 -> Switch2/3
  Eff Map/1 -> Gain1/1
  Abs/1 -> Eff Map/1
  Gain1/1 -> Math Function/1
  Math Function/1 -> Eff2k/1, Product4/2
  Product4/1 -> MotPwrElecReq/1
  Abs1/1 -> Eff Map/2
  rads_to_rpm/1 -> Abs/1
  Product/1 -> Switch2/2
  MotSpd/1 -> Product3/1, Product/1, rads_to_rpm/1
  MotTrqCmd/1 -> Product3/2, Product/2, Abs1/1

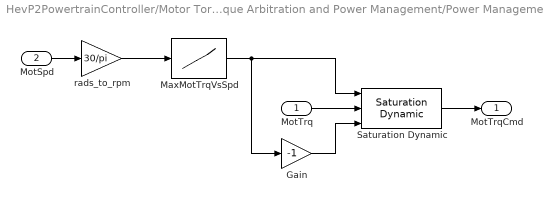
== system HevP2PowertrainController/Motor Torque Arbitration and Power Management/Power Management/Torque Limit ==
  MotTrq : Inport
  MotSpd : Inport  Port=2
  Gain : Gain  Gain=-1
  MaxMotTrqVsSpd : Lookup_n-D  NumberOfTableDimensions=1  BreakpointsForDimension1=w_eff_bp  Table=MotTrq  ExtrapMethod=Clip  UseLastTableValue=on  InternalRulePriority=Speed  OutDataTypeStr=Inherit: Inherit from 'Table data'  RndMeth=Simplest
  Saturation Dynamic : simulink/Discontinuities/Saturation Dynamic  OutMin=[]  OutMax=[]  OutDataTypeStr=Inherit: Same as second input  OutDataType=fixdt(1, 16)  OutScaling=2^-10  DoSatur=off
  rads_to_rpm : Gain  Gain=30/pi
  MotTrqCmd : Outport  VectorParamsAs1DForOutWhenUnconnected=off
  wires:
  MotTrq/1 -> Saturation Dynamic/2
  Saturation Dynamic/1 -> MotTrqCmd/1
  MotSpd/1 -> rads_to_rpm/1
  MaxMotTrqVsSpd/1 -> Gain/1, Saturation Dynamic/1
  rads_to_rpm/1 -> MaxMotTrqVsSpd/1
  Gain/1 -> Saturation Dynamic/3
